simulink model "zaw_state"  (R2013a)
settings: Solver=ode3  StartTime=0.0  StopTime=50.0  FixedStep=0.005  RelTol=1e-3
values from neighbouring files (symbols this model uses):
  A = [0 0 -4500 58.3333333333 0 0 388.888888889 -58.3333333333 1 0 -23.3333333333 3.33333333333 ... (16 elements, 4x4)]    [matlab1.mat]    (also in matlab3.mat; matlab4.mat = [0 0 -4222.22222222 16.6666666667 0 0 111.111111111 -16.6666; refsstat.m = [0 0 1 0;0 0 0 1;-(k1+k2)/m1 k2/m1 -(c1+c2)/m1 c2/m1; k2/m2 )
  B = [1.11111111111 0 4137.03703704 3.7037037037]    [matlab1.mat]    (also in matlab3.mat; matlab4.mat; refsstat.m = [c1/m1;0;c1*(c1+c2)/(m1*m1)+k1/m1;c1*c2/(m1*m2)])
  C = [0 1 0 0]    [matlab1.mat]    (also in matlab3.mat; matlab4.mat)
  D = 0    [matlab1.mat]    (also in matlab3.mat; matlab4.mat)
settings Model: Creator=adasdeb  LastModifiedBy=adasdeb

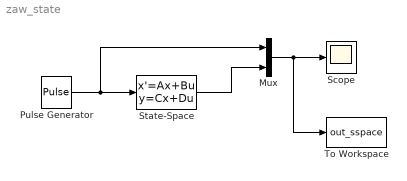
== system zaw_state ==
  Mux : Mux  Inputs=2
  Pulse Generator : DiscretePulseGenerator  PulseType=Time based  Period=0.1  PulseWidth=50
  Scope : Scope
      settings: YMin=-3  YMax=3
  State-Space : StateSpace  A=A  B=B  C=C  D=D
  To Workspace : ToWorkspace  VariableName=out_sspace  SampleTime=-1
  wires:
  Pulse Generator/1 -> Mux/1, State-Space/1
  State-Space/1 -> Mux/2
  Mux/1 -> To Workspace/1, Scope/1
